simulink model "complementray_filter"  (R2024b)
settings: Solver=FixedStepAuto  StartTime=0.0  StopTime=10.0  FixedStep=0.01  RelTol=1e-3
settings Model: Creator=ARULPAVALAN S A  LastModifiedBy=ARULPAVALAN S A

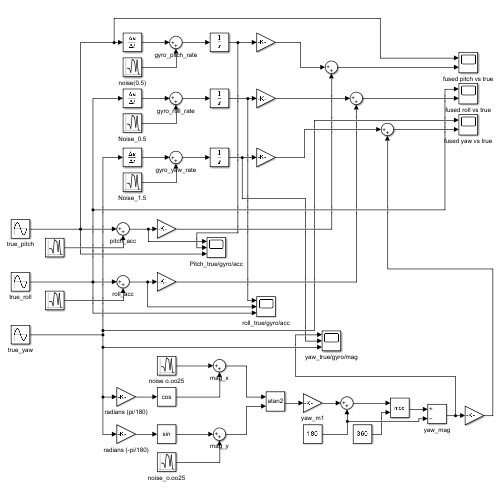
[thumbnail: Simulink's stored preview of the top-level diagram]
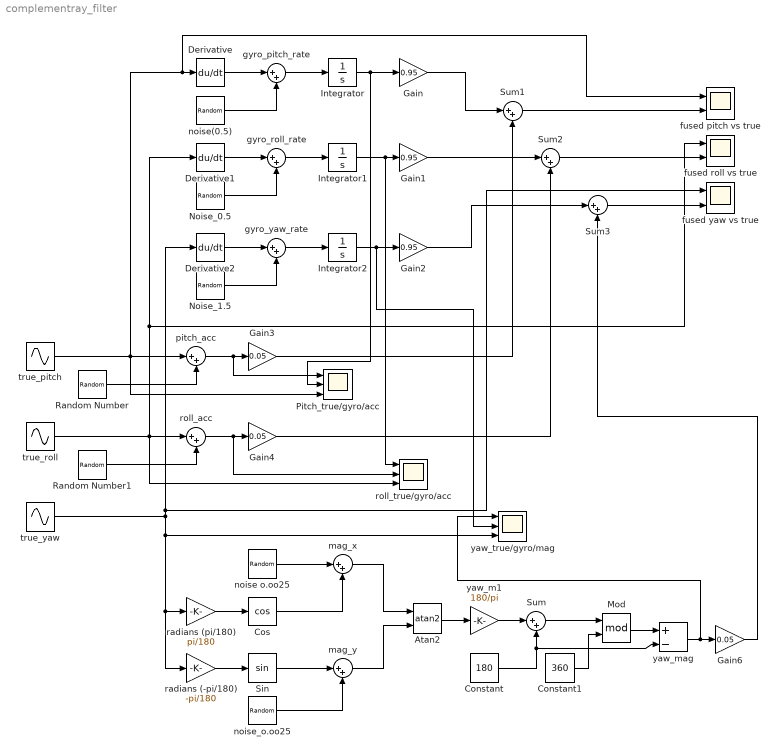
== system complementray_filter ==
  Atan2 : Trigonometry  Operator=atan2
  Constant : Constant  Value=180
  Constant1 : Constant  Value=360
  Cos : Trigonometry  Operator=cos
  Derivative : Derivative
  Derivative1 : Derivative
  Derivative2 : Derivative
  Gain : Gain  Gain=0.95
  Gain1 : Gain  Gain=0.95
  Gain2 : Gain  Gain=0.95
  Gain3 : Gain  Gain=0.05
  Gain4 : Gain  Gain=0.05
  Gain6 : Gain  Gain=0.05
  Integrator : Integrator
  Integrator1 : Integrator
  Integrator2 : Integrator
  Mod : Math  Operator=mod
  Noise_0.5 : RandomNumber  Variance=0.25  SampleTime=0.1
  Noise_1.5 : RandomNumber  Variance=2.25  SampleTime=0.1
  Pitch_true/gyro/acc : Scope  NumInputPorts=3
  Random Number : RandomNumber  Variance=2.25  SampleTime=0.1
  Random Number1 : RandomNumber  Variance=2.25  SampleTime=0.1
  Sin : Trigonometry
  Sum{,1..3} (4 alike) : Sum  Inputs=|++
  fused pitch vs true : Scope  NumInputPorts=2
  fused roll vs true : Scope  NumInputPorts=2
  fused yaw vs true : Scope  NumInputPorts=2
  "gyro_pitch_rate " : Sum  Inputs=|++
  "gyro_roll_rate " : Sum  Inputs=|++
  "gyro_yaw_rate " : Sum  Inputs=|++
  mag_x : Sum  Inputs=|++
  mag_y : Sum  Inputs=|++
  noise o.oo25 : RandomNumber  Variance=0.0025  SampleTime=0.1
  noise(0.5) : RandomNumber  Variance=0.25  SampleTime=0.1
  noise_o.oo25 : RandomNumber  Variance=0.0025  SampleTime=0.1
  pitch_acc : Sum  Inputs=|++
  radians (-pi/180) : Gain  Gain=-pi/180
  radians (pi/180) : Gain  Gain=pi/180
  roll_acc : Sum  Inputs=|++
  roll_true/gyro/acc : Scope  NumInputPorts=3
  true_pitch : Sin  Amplitude=10  Frequency=0.6283  SampleTime=0
  true_roll : Sin  Amplitude=5  Frequency=0.3142  SampleTime=0
  true_yaw : Sin  Amplitude=45  Frequency=0.1257  SampleTime=0
  yaw_m1 : Gain  Gain=180/pi
  yaw_mag : Sum  Inputs=+-
  yaw_true/gyro/mag : Scope  NumInputPorts=3
  wires:
  true_yaw/1 -> fused yaw vs true/1, Derivative2/1, yaw_true/gyro/mag/3, radians (-pi/180)/1, radians (pi/180)/1
  true_roll/1 -> roll_true/gyro/acc/3, fused roll vs true/1, Derivative1/1, roll_acc/1
  true_pitch/1 -> Pitch_true/gyro/acc/3, fused pitch vs true/1, Derivative/1, pitch_acc/1
  Random Number/1 -> pitch_acc/2
  Random Number1/1 -> roll_acc/2
  Derivative/1 -> "gyro_pitch_rate "/1
  noise(0.5)/1 -> "gyro_pitch_rate "/2
  Derivative1/1 -> "gyro_roll_rate "/1
  Noise_0.5/1 -> "gyro_roll_rate "/2
  Noise_1.5/1 -> "gyro_yaw_rate "/2
  Derivative2/1 -> "gyro_yaw_rate "/1
  radians (pi/180)/1 -> Cos/1
  radians (-pi/180)/1 -> Sin/1
  noise o.oo25/1 -> mag_x/1
  Cos/1 -> mag_x/2
  Sin/1 -> mag_y/1
  noise_o.oo25/1 -> mag_y/2
  mag_x/1 -> Atan2/1
  mag_y/1 -> Atan2/2
  Atan2/1 -> yaw_m1/1
  yaw_m1/1 -> Sum/1
  Constant/1 -> Sum/2, yaw_mag/2
  Sum/1 -> Mod/1
  Constant1/1 -> Mod/2
  Mod/1 -> yaw_mag/1
  "gyro_pitch_rate "/1 -> Integrator/1
  Integrator/1 -> Pitch_true/gyro/acc/2, Gain/1
  Integrator1/1 -> roll_true/gyro/acc/1, Gain1/1
  "gyro_roll_rate "/1 -> Integrator1/1
  Integrator2/1 -> yaw_true/gyro/mag/2, Gain2/1
  "gyro_yaw_rate "/1 -> Integrator2/1
  roll_acc/1 -> roll_true/gyro/acc/2, Gain4/1
  pitch_acc/1 -> Pitch_true/gyro/acc/1, Gain3/1
  Gain/1 -> Sum1/1
  Gain3/1 -> Sum1/2
  Gain4/1 -> Sum2/2
  Gain1/1 -> Sum2/1
  Gain2/1 -> Sum3/1
  yaw_mag/1 -> yaw_true/gyro/mag/1, Gain6/1
  Gain6/1 -> Sum3/2
  Sum1/1 -> fused pitch vs true/2
  Sum2/1 -> fused roll vs true/2
  Sum3/1 -> fused yaw vs true/2
